simulink model "dssbpsk"  (R2015a)
settings: Solver=ode45  StartTime=0.0  StopTime=10.0  RelTol=1e-3
libraries: commchan3 x1, commsink2 x1, commfilt2 x1, commanapbnd3 x1, commrandsrc2 x1
settings Model: Creator=Sonu Sharma  LastModifiedBy=Sonu Sharma

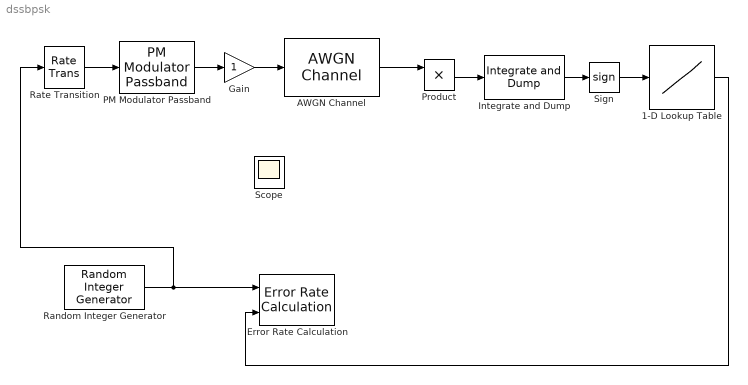
== system dssbpsk ==
  1-D Lookup Table : Lookup_n-D  NumberOfTableDimensions=1  BreakpointsForDimension1=[-5:5]  Table=tanh([-5:5])  InternalRulePriority=Speed  RndMeth=Simplest  InputSameDT=on
  AWGN Channel : commchan3/AWGN Channel  InputProcessing=Columns as channels (frame based)  seed=67  noiseMode="Signal to noise ratio  (Eb/No)"  EbNodB=10  EsNodB=10  SNRdB=10  bitsPerSym=1  Ps=1  Tsym=1  variance=1
  Error Rate Calculation : commsink2/Error Rate Calculation  N=0  st_delay=0  cp_mode=Entire frame  subframe=[]  PMode=Workspace  WsName=ErrorVec  RsMode2=off  stop=off  numErr=100  maxBits=1e6
  Gain : Gain
  Integrate and Dump : commfilt2/Integrate and Dump  obssamples=8  offsetsamples=0  nodump=off  roundingMode=Floor  overflowMode=off
  PM Modulator Passband : commanapbnd3/PM Modulator Passband  Fc=300  Ph=0  Kc=pi/2
  Product : Product
  Random Integer Generator : commrandsrc2/Random Integer Generator  mul=8  seed=37  Ts=1  frameBased=off  sampPerFrame=1  orient=off  outDataType=double
  Rate Transition : RateTransition
  Scope : Scope
  Sign : Signum
  wires:
  Random Integer Generator/1 -> Rate Transition/1, Error Rate Calculation/1
  Rate Transition/1 -> PM Modulator Passband/1
  PM Modulator Passband/1 -> Gain/1
  Gain/1 -> AWGN Channel/1
  AWGN Channel/1 -> Product/1
  Product/1 -> Integrate and Dump/1
  Integrate and Dump/1 -> Sign/1
  Sign/1 -> 1-D Lookup Table/1
  1-D Lookup Table/1 -> Error Rate Calculation/2
